simulink model "Projet_Placement_PZ_sim_LIMA_MILITAO_PINHEIRO"  (R2019a)
settings: Solver=VariableStepAuto  StartTime=0.0  StopTime=10.0  FixedStep=1e-6  RelTol=1e-3
undefined symbols (not defined in the file): Am_omega, Bm_omega, den, K_den_PP, K_num_PP, numG2, Te, tsim
settings Model: Creator=dougl  LastModifiedBy=dougl
settings DebuggingCC: UnconnectedInputMsg=none  UnconnectedOutputMsg=none  UnconnectedLineMsg=none  SFMachineParentedDataDiag=error

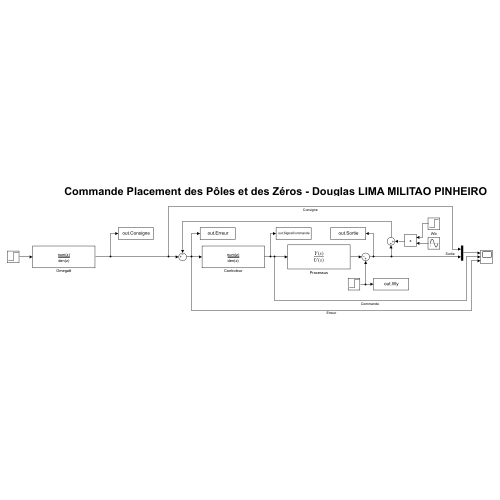
[thumbnail: Simulink's stored preview of the top-level diagram]
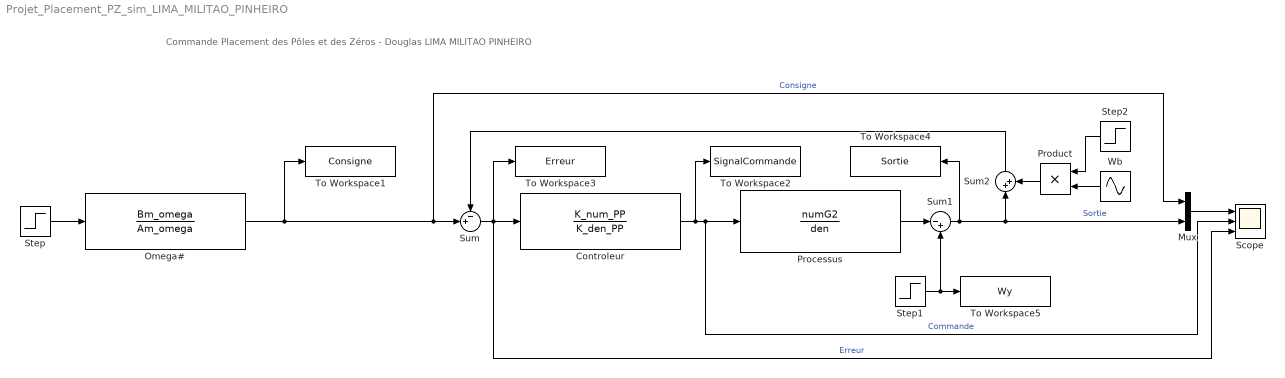
== system Projet_Placement_PZ_sim_LIMA_MILITAO_PINHEIRO ==
  note: Commande Placement des Pôles et des Zéros - Douglas LIMA MILITAO PINHEIRO
  Controleur : DiscreteFilter  Numerator=K_num_PP  Denominator=K_den_PP  SampleTime=Te
  Mux : Mux  Inputs=2
  Omega# : DiscreteFilter  Numerator=Bm_omega  Denominator=Am_omega  SampleTime=Te
  Processus : TransferFcn  Numerator=numG2  Denominator=den
  Product : Product
  Scope : Scope  NumInputPorts=3
  Step : Step  After=5  SampleTime=0
  Step1 : Step  Time=5  After=15  SampleTime=0
  Step2 : Step  Time=7  SampleTime=0
  Sum : Sum  Inputs=-+|
  Sum1 : Sum  Inputs=|-+
  Sum2 : Sum  Inputs=|++
  To Workspace1 : ToWorkspace  VariableName=Consigne  SampleTime=tsim
  To Workspace2 : ToWorkspace  VariableName=SignalCommande  SampleTime=tsim
  To Workspace3 : ToWorkspace  VariableName=Erreur  SampleTime=tsim
  To Workspace4 : ToWorkspace  VariableName=Sortie  SampleTime=tsim
  To Workspace5 : ToWorkspace  VariableName=Wy  SampleTime=tsim
  Wb : Sin  Amplitude=3  Frequency=2*pi*10  SampleTime=0
  wires:
  Sum1/1 -> Sum2/1, Mux/2, To Workspace4/1  "Sortie"
  Sum/1 -> Scope/3, To Workspace3/1, Controleur/1  "Erreur"
  Step/1 -> Omega#/1
  Omega#/1 -> To Workspace1/1, Sum/2, Mux/1  "Consigne"
  Processus/1 -> Sum1/1
  Step1/1 -> To Workspace5/1, Sum1/2
  Controleur/1 -> Scope/2, Processus/1, To Workspace2/1  "Commande"
  Mux/1 -> Scope/1
  Step2/1 -> Product/1
  Product/1 -> Sum2/2
  Wb/1 -> Product/2
  Sum2/1 -> Sum/1
